simulink model "QAM8"  (Simulink 7.5)
settings: Solver=ode45  StartTime=0.0  StopTime=inf  RelTol=1e-3
InitFcn:
  | wt = 0:2*pi/30:4*pi;   % time axis for pulse generation
  | 
  | g = rcosine(1,10);      % raised cosine as chosen pulse
  | 
  | inphase_pulse = g .* cos(wt);      % in-phase pulse
  | quadrature_pulse = g .* sin(wt);   % quadrature pulse
undefined symbols (not defined in the file or in its folder): get
libraries: commsink2 x3, simulink x2, commdigbbndam2 x2, commchan3 x1, commrandsrc2 x1
settings Model: Creator=Pc_sary  LastModifiedBy=Pc_sary
settings OptimizationCC: InlineInvariantSignals=on  InitFltsAndDblsToZero=on
settings DebuggingCC: SaveWithParameterizedLinksMsg=none  SignalResolutionControl=TryResolveAllWithWarning  MultiTaskDSMMsg=warning  MultiTaskCondExecSysMsg=none  StrictBusMsg=None
settings RTWCC: IncludeERTFirstTime=on
settings GRTTargetCC: TargetFcnLib=ansi_tfl_tmw.mat

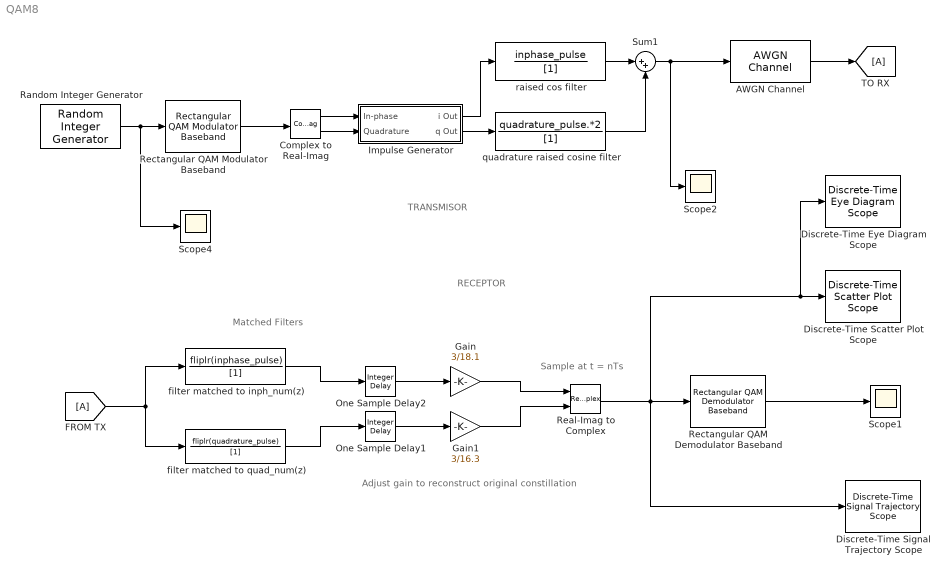
== system QAM8 ==
  note: TRANSMISOR
  note: RECEPTOR
  note: Matched Filters
  note: Adjust gain to reconstruct
      | original constillation
  note: Sample at t = nTs
  AWGN Channel : commchan3/AWGN Channel  SystemSampleTime=-1  seed=67  noiseMode="Signal to noise ratio  (Eb/No)"  EbNodB=7  EsNodB=10  SNRdB=10  bitsPerSym=1  Ps=1  Tsym=1  variance=1
  Complex to Real-Imag : ComplexToRealImag
  Discrete-Time Eye Diagram Scope : commsink2/Discrete-Time Eye Diagram Scope  Tag=EyeDiagram  SystemSampleTime=-1  sampPerSymb=8  offsetEye=0  symbPerTrace=1  numTraces=40  numNewFrames=10  LineStyles=-  LineColors=b  dupPoints=on  fading=on  render=on  AxisGrid=on  yMin=-3.7985824914649  yMax=3.73873679764653  inphaseLabel=In-phase Amplitude  quadratureLabel=Quadrature Amplitude  openScopeAtSimStart=on  dispDiagram=In-phase and Quadrature  FrameNumber=off  FigPos=[296 120 560 644]  figTitle=Eye Diagram  block_type_=eye  numLinesMax=8
  Discrete-Time Scatter Plot Scope : commsink2/Discrete-Time Scatter Plot Scope  Tag=ScatterPlot  SystemSampleTime=-1  sampPerSymb=1  offsetEye=0  numTraces=40  numNewFrames=10  LineMarkers=.  LineColors=b  fading=on  render=on  AxisGrid=on  xMin=-4.96054901766682  xMax=4.98260094663848  yMin=-4.96005977321457  yMax=4.98309019109073  inphaseLabel=In-phase Amplitude  quadratureLabel=Quadrature Amplitude  openScopeAtSimStart=on  FrameNumber=off  FigPos=[296 204 560 560]  figTitle=Scatter Plot  numLinesMax=8  block_type_=scatter
  Discrete-Time Signal Trajectory Scope : commsink2/Discrete-Time Signal Trajectory Scope  Tag=SignalTrajectory  SystemSampleTime=-1  sampPerSymb=8  offsetEye=0  numTraces=40  numNewFrames=10  LineStyles=-  LineColors=b  fading=on  render=on  AxisGrid=on  xMin=-3.3  xMax=3.315  yMin=-3.3  yMax=3.315  inphaseLabel=In-phase Amplitude  quadratureLabel=Quadrature Amplitude  openScopeAtSimStart=on  FrameNumber=off  FigPos=get(0,'defaultfigureposition');  figTitle=Signal Trajectory  numLinesMax=8  block_type_=xy
  Gain : Gain  Gain=3/18.1  ParameterDataType=sfix(16)  ParameterScaling=2^0  OutDataType=sfix(16)  OutScaling=2^0
  Gain1 : Gain  Gain=3/16.3  ParameterDataType=sfix(16)  ParameterScaling=2^0  OutDataType=sfix(16)  OutScaling=2^0
  Impulse Generator : Subsystem
  One Sample Delay1 : simulink/Discrete/Integer Delay  vinit=0.0  samptime=-1  NumDelays=1
  One Sample Delay2 : simulink/Discrete/Integer Delay  vinit=0.0  samptime=-1  NumDelays=1
  Random Integer Generator : commrandsrc2/Random Integer Generator  SystemSampleTime=-1  mul=8  seed=37  Ts=length(wt)  frameBased=off  sampPerFrame=1  orient=off  outDataType=double
  Real-Imag to Complex : RealImagToComplex  SampleTime=length(wt)
  Rectangular QAM Demodulator Baseband : commdigbbndam2/Rectangular QAM Demodulator Baseband  M=8  OutType=Integer  Dec=Binary  PowType=Min. distance between symbols  MinDist=2  AvgPow=1  PeakPow=1  Ph=0  numSamp=1
  Rectangular QAM Modulator Baseband : commdigbbndam2/Rectangular QAM Modulator Baseband  M=8  InType=Integer  Enc=Binary  PowType=Min. distance between symbols  MinDist=2  AvgPow=1  PeakPow=1  Ph=0  numSamp=1
  Scope1 : Scope
      settings: TimeRange=1000  YMin=0  YMax=15
  Scope2 : Scope
      settings: TimeRange=1000
  Scope4 : Scope
      settings: TimeRange=1000  YMin=0  YMax=15  SaveName=ScopeData3
  Sum1 : Sum  Inputs=|++  OutDataType=sfix(16)  OutScaling=2^0
  filter matched to inph_num(z) : DiscreteFilter  Numerator=fliplr(inphase_pulse)  Denominator=[1]  SampleTime=1
  filter matched to quad_num(z) : DiscreteFilter  Numerator=fliplr(quadrature_pulse)  Denominator=[1]  SampleTime=1
  quadrature raised cosine filter : DiscreteFilter  Numerator=quadrature_pulse.*2  Denominator=[1]  SampleTime=1
  raised cos filter : DiscreteFilter  Numerator=inphase_pulse  Denominator=[1]  SampleTime=1
  wires:
  Rectangular QAM Modulator Baseband/1 -> Complex to Real-Imag/1
  quadrature raised cosine filter/1 -> Sum1/2
  raised cos filter/1 -> Sum1/1
  Complex to Real-Imag/1 -> Impulse Generator/1(In-phase)
  Complex to Real-Imag/2 -> Impulse Generator/2(Quadrature)
  Impulse Generator/1(i Out) -> raised cos filter/1
  Impulse Generator/2(q Out) -> quadrature raised cosine filter/1
  [A] -> filter matched to quad_num(z)/1, filter matched to inph_num(z)/1
  filter matched to inph_num(z)/1 -> One Sample Delay2/1
  filter matched to quad_num(z)/1 -> One Sample Delay1/1
  One Sample Delay2/1 -> Gain/1
  One Sample Delay1/1 -> Gain1/1
  Sum1/1 -> AWGN Channel/1, Scope2/1
  AWGN Channel/1 -> [A]
  Random Integer Generator/1 -> Rectangular QAM Modulator Baseband/1, Scope4/1
  Gain/1 -> Real-Imag to Complex/1
  Gain1/1 -> Real-Imag to Complex/2
  Rectangular QAM Demodulator Baseband/1 -> Scope1/1
  Real-Imag to Complex/1 -> Rectangular QAM Demodulator Baseband/1, Discrete-Time Scatter Plot Scope/1, Discrete-Time Eye Diagram Scope/1, Discrete-Time Signal Trajectory Scope/1

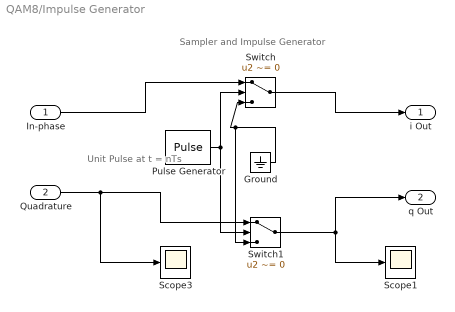
== system QAM8/Impulse Generator ==
  note: Unit Pulse
      | at t = nTs
  note: Sampler and Impulse Generator
  In-phase : Inport  OutDataType=sfix(16)  OutScaling=2^0
  Quadrature : Inport  Port=2  OutDataType=sfix(16)  OutScaling=2^0
  Ground : Ground
  Pulse Generator : DiscretePulseGenerator  Amplitude=1  Period=length(wt)  PulseWidth=1  PhaseDelay=0  SampleTime=1
  Scope1 : Scope
      settings: TimeRange=1000  SaveName=ScopeData4
  Scope3 : Scope
      settings: TimeRange=1000  SaveName=ScopeData2
  Switch : Switch  Criteria=u2 ~= 0
  Switch1 : Switch  Criteria=u2 ~= 0
  i Out : Outport  OutDataType=sfix(16)  OutScaling=2^0
  q Out : Outport  Port=2  OutDataType=sfix(16)  OutScaling=2^0
  wires:
  Pulse Generator/1 -> Switch/2, Switch1/2
  Ground/1 -> Switch/3, Switch1/3
  In-phase/1 -> Switch/1
  Quadrature/1 -> Switch1/1, Scope3/1
  Switch/1 -> i Out/1
  Switch1/1 -> q Out/1, Scope1/1
